simulink model "DEF_IEEE14_case1"  (R2023b)
settings: Solver=FixedStepAuto  StartTime=0  StopTime=80  FixedStep=Ts  RelTol=1e-3
StopFcn:
  | %data_idq_all = out.data_idq_all;
  | %save('Oscillation_July\data\data_idq_all.mat','data_idq_all');
  | %data_vdq_all = out.data_vdq_all;
  | %save('Oscillation_July\data\data_vdq_all.mat','data_vdq_all');
values from neighbouring files (symbols this model uses):
  freq_sel = imag(Mode_Hz)    [Mode_Right_Eig.m]
  Mode_Rad = D(ModeSel, ModeSel)    [Mode_Right_Eig.m]
undefined symbols (not defined in the file or in its folder): ApparatusDiscreDamping, ApparatusPara, ApparatusPowerFlow, ApparatusType, DiscIntNeverNeededParam, Fbase, fpll, k_lpf, lpf_A, lpf_B, lpf_C, lpf_D, OtherInputs, Sbase, Tdef_start, Ts, Vbase, Wbase, wc_lpf, x_e, Ybase, Zbase
libraries: spsFourierLib x50, SimplusGT x46, spsGroundLib x22, spsThreePhaseSeriesRLCBranchLib x20, spsThreePhaseParallelRLCBranchLib x14, spsThreePhaseTransformerTwoWindingsLib x3, eeGeneralControl x2, spspowerguiLib x1
(part 2 of 3)

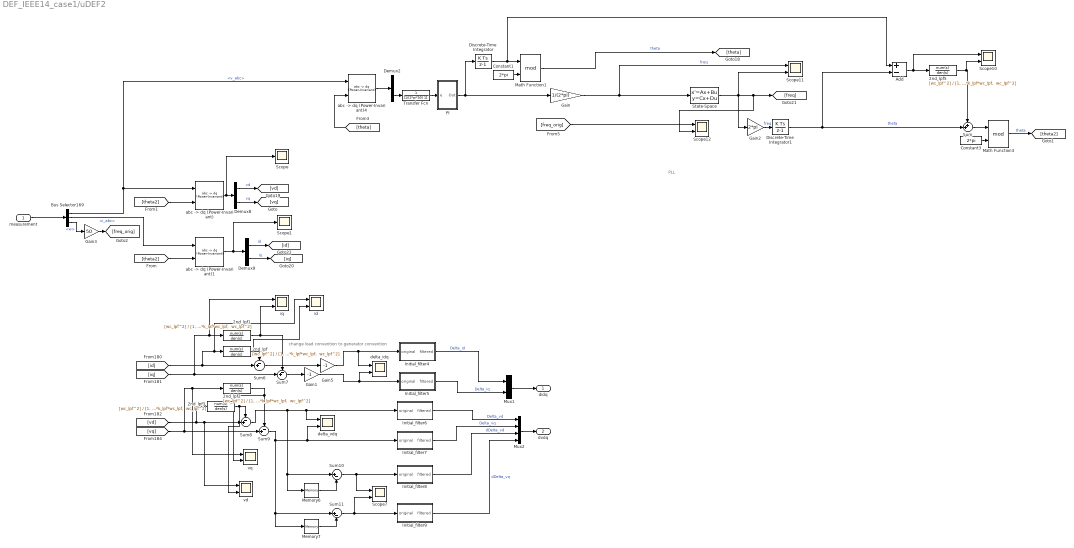
== system DEF_IEEE14_case1/uDEF2 ==
  note: change load convention to generator convention
  note: PLL
  measurement : Inport
  2nd_lpf{,1..3,5} (5 alike) : TransferFcn  Numerator=[wc_lpf^2]  Denominator="[1, 2*k_lpf*wc_lpf,  wc_lpf^2]"
  Add : Sum  Inputs=+-
  Bus Selector169 : BusSelector  OutputSignals=v_abc,i_abc,w
  Constant1 : Constant  Value=2*pi
  Constant3 : Constant  Value=2*pi
  Demux2 : Demux  Outputs=2
  Demux8 : Demux  Outputs=2
  Demux9 : Demux  Outputs=2
  Discrete-Time Integrator : DiscreteIntegrator  SampleTime=Ts  ICPrevOutput=DiscIntNeverNeededParam  ICPrevScaledInput=DiscIntNeverNeededParam
  Discrete-Time Integrator1 : DiscreteIntegrator  SampleTime=Ts  ICPrevOutput=DiscIntNeverNeededParam  ICPrevScaledInput=DiscIntNeverNeededParam
  Gain : Gain  Gain=1/(2*pi)
  Gain1 : Gain  Gain=-1
  Gain2 : Gain  Gain=2*pi
  Gain3 : Gain  Gain=50
  Gain5 : Gain  Gain=-1
  Initial_filter4 : Subsystem
  Initial_filter5 : Subsystem
  Initial_filter6 : Subsystem
  Initial_filter7 : Subsystem
  Initial_filter8 : Subsystem
  Initial_filter9 : Subsystem
  Math Function1 : Math  Operator=mod  SignedPower=on
  Math Function3 : Math  Operator=mod  SignedPower=on
  Memory6 : Memory
  Memory7 : Memory
  Mux1 : Mux  Inputs=2
  Mux2 : Mux
  PI : Subsystem  mask{Kp_PLL=2*pi*fpll, Ki_PLL=(2*pi*fpll)^2/4, IntSat_PLL=20000}
      mask prompts: Kp_PLL "Proportional (P)"; Ki_PLL "Integral (I)"; IntSat_PLL "Integrator Saturation Limit"
      mask DialogControl DescGroupVar Prompt: PLL Parameters
  Scope : Scope
  Scope1 : Scope
  Scope{7,10..12} (4 alike) : Scope  NumInputPorts=2
  State-Space : StateSpace  A=lpf_A  B=lpf_B  C=lpf_C  D=lpf_D  InitialCondition=[0,50/lpf_C(2)]
  Sum : Sum  Inputs=++|
  Sum10 : Sum  Inputs=|+-
  Sum11 : Sum  Inputs=|+-
  Sum{6..9} (4 alike) : Sum  Inputs=-+|
  Transfer Fcn : TransferFcn  Denominator=[1/(2*pi*50) 1]
  "abc -> dq (Power-Invariant)" : SimplusGT/abc -> dq (Power-Invariant)  SystemSampleTime=-1  VariantActivationTime=update diagram  AllowFlexibleInterface=on  Latency=0  AutoFrameSizeCalculation=off
      settings: SourceProductName=Simplus Grid Tool
  "abc -> dq (Power-Invariant)1" : SimplusGT/abc -> dq (Power-Invariant)  SystemSampleTime=-1  VariantActivationTime=update diagram  AllowFlexibleInterface=on  Latency=0  AutoFrameSizeCalculation=off
      settings: SourceProductName=Simplus Grid Tool
  "abc -> dq (Power-Invariant)4" : SimplusGT/abc -> dq (Power-Invariant)  SystemSampleTime=-1  VariantActivationTime=update diagram  AllowFlexibleInterface=on  Latency=0  AutoFrameSizeCalculation=off
      settings: SourceProductName=Simplus Grid Tool
  delta_idq : Scope  NumInputPorts=2
  delta_vdq : Scope  NumInputPorts=2
  id : Scope  NumInputPorts=2
  iq : Scope  NumInputPorts=2
  vd : Scope  NumInputPorts=2
  vq : Scope  NumInputPorts=2
  didq : Outport
  dvdq : Outport  Port=2
  wires:
  [vq] -> vq/1, 2nd_lpf2/1, Sum9/2
  Sum11/1 -> Scope7/2, Initial_filter9/1(original)
  Sum6/1 -> Gain5/1
  "abc -> dq (Power-Invariant)1"/1 -> Scope1/1, Demux9/1
  [theta2] -> "abc -> dq (Power-Invariant)1"/2
  Sum9/1 -> Memory7/1, Sum11/1, delta_vdq/2, Initial_filter7/1(original)
  [vd] -> 2nd_lpf3/1, vd/1, Sum8/2
  Demux9/1 -> [id]  "id"
  Sum8/1 -> Memory6/1, Sum10/1, delta_vdq/1, Initial_filter6/1(original)
  Initial_filter7/1(filtered) -> Mux2/2  "Delta_vq"
  Bus Selector169/1 -> "abc -> dq (Power-Invariant)4"/1, "abc -> dq (Power-Invariant)"/1  "<v_abc>"
  Demux9/2 -> [iq]  "iq"
  [id] -> id/1, 2nd_lpf/1, Sum6/2
  2nd_lpf/1 -> id/2, Sum6/1
  Sum10/1 -> Scope7/1, Initial_filter8/1(original)
  Memory7/1 -> Sum11/2
  Initial_filter9/1(filtered) -> Mux2/4  "dDelta_vq"
  2nd_lpf1/1 -> iq/2, Sum7/1
  Mux1/1 -> didq/1
  Memory6/1 -> Sum10/2
  Bus Selector169/2 -> "abc -> dq (Power-Invariant)1"/1  "<i_abc>"
  Sum7/1 -> Gain1/1
  Demux8/1 -> [vd]  "vd"
  Initial_filter6/1(filtered) -> Mux2/1  "Delta_vd"
  Initial_filter5/1(filtered) -> Mux1/2  "Delta_iq"
  Mux2/1 -> dvdq/1
  [iq] -> iq/1, 2nd_lpf1/1, Sum7/2
  Initial_filter4/1(filtered) -> Mux1/1  "Delta_id"
  2nd_lpf2/1 -> Sum9/1, vq/2
  Gain1/1 -> delta_idq/2, Initial_filter5/1(original)
  Demux8/2 -> [vq]  "vq"
  "abc -> dq (Power-Invariant)"/1 -> Scope/1, Demux8/1
  Initial_filter8/1(filtered) -> Mux2/3  "dDelta_vd"
  [theta2] -> "abc -> dq (Power-Invariant)"/2
  2nd_lpf3/1 -> vd/2, Sum8/1
  Gain5/1 -> delta_idq/1, Initial_filter4/1(original)
  [theta] -> "abc -> dq (Power-Invariant)4"/2
  Constant1/1 -> Math Function1/2
  Add/1 -> 2nd_lpf5/1, Scope10/1
  Discrete-Time Integrator/1 -> Math Function1/1, Add/1
  Gain2/1 -> Discrete-Time Integrator1/1  "freq"
  "abc -> dq (Power-Invariant)4"/1 -> Demux2/1
  Transfer Fcn/1 -> PI/1(e)
  Math Function1/1 -> [theta]  "theta"
  Gain/1 -> State-Space/1, Scope11/1  "freq"
  PI/1(Out) -> Gain/1, Discrete-Time Integrator/1
  Demux2/2 -> Transfer Fcn/1
  [freq_orig] -> Scope12/1
  Math Function3/1 -> [theta2]  "theta"
  2nd_lpf5/1 -> Sum/1, Scope10/2
  Sum/1 -> Math Function3/1
  State-Space/1 -> Scope12/2, [freq], Scope11/2, Gain2/1
  Constant3/1 -> Math Function3/2
  Discrete-Time Integrator1/1 -> Add/2, Sum/2  "theta"
  measurement/1 -> Bus Selector169/1
  Gain3/1 -> [freq_orig]
  Bus Selector169/3 -> Gain3/1  "<w>"

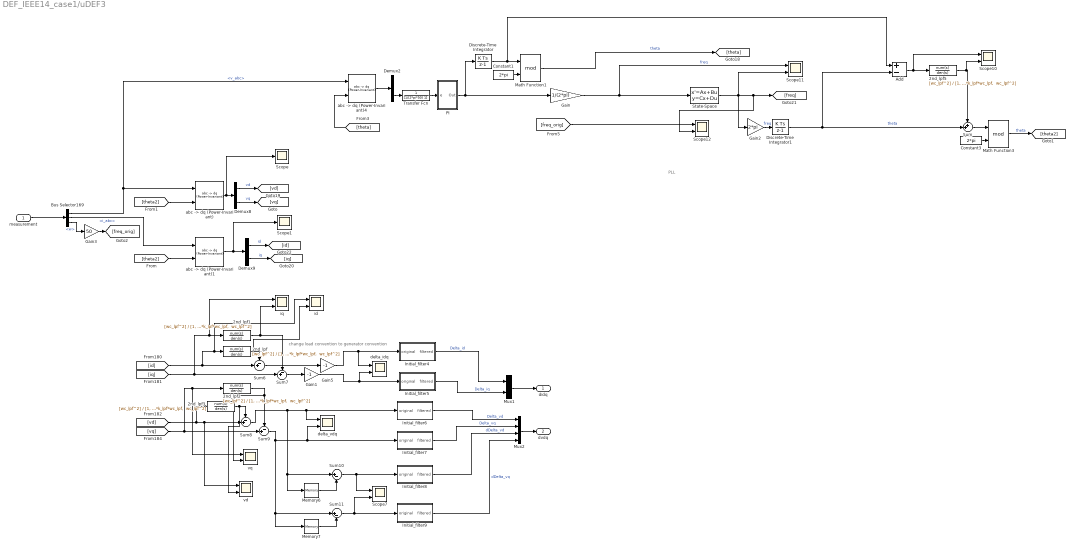
== system DEF_IEEE14_case1/uDEF3 ==
  note: PLL
  note: change load convention to generator convention
  measurement : Inport
  2nd_lpf{,1..3,5} (5 alike) : TransferFcn  Numerator=[wc_lpf^2]  Denominator="[1, 2*k_lpf*wc_lpf,  wc_lpf^2]"
  Add : Sum  Inputs=+-
  Bus Selector169 : BusSelector  OutputSignals=v_abc,i_abc,w
  Constant1 : Constant  Value=2*pi
  Constant3 : Constant  Value=2*pi
  Demux2 : Demux  Outputs=2
  Demux8 : Demux  Outputs=2
  Demux9 : Demux  Outputs=2
  Discrete-Time Integrator : DiscreteIntegrator  SampleTime=Ts  ICPrevOutput=DiscIntNeverNeededParam  ICPrevScaledInput=DiscIntNeverNeededParam
  Discrete-Time Integrator1 : DiscreteIntegrator  SampleTime=Ts  ICPrevOutput=DiscIntNeverNeededParam  ICPrevScaledInput=DiscIntNeverNeededParam
  Gain : Gain  Gain=1/(2*pi)
  Gain1 : Gain  Gain=-1
  Gain2 : Gain  Gain=2*pi
  Gain3 : Gain  Gain=50
  Gain5 : Gain  Gain=-1
  Initial_filter4 : Subsystem
  Initial_filter5 : Subsystem
  Initial_filter6 : Subsystem
  Initial_filter7 : Subsystem
  Initial_filter8 : Subsystem
  Initial_filter9 : Subsystem
  Math Function1 : Math  Operator=mod  SignedPower=on
  Math Function3 : Math  Operator=mod  SignedPower=on
  Memory6 : Memory
  Memory7 : Memory
  Mux1 : Mux  Inputs=2
  Mux2 : Mux
  PI : Subsystem  mask{Kp_PLL=2*pi*fpll, Ki_PLL=(2*pi*fpll)^2/4, IntSat_PLL=20000}
      mask prompts: Kp_PLL "Proportional (P)"; Ki_PLL "Integral (I)"; IntSat_PLL "Integrator Saturation Limit"
      mask DialogControl DescGroupVar Prompt: PLL Parameters
  Scope : Scope
  Scope1 : Scope
  Scope{7,10..12} (4 alike) : Scope  NumInputPorts=2
  State-Space : StateSpace  A=lpf_A  B=lpf_B  C=lpf_C  D=lpf_D  InitialCondition=[0,50/lpf_C(2)]
  Sum : Sum  Inputs=++|
  Sum10 : Sum  Inputs=|+-
  Sum11 : Sum  Inputs=|+-
  Sum{6..9} (4 alike) : Sum  Inputs=-+|
  Transfer Fcn : TransferFcn  Denominator=[1/(2*pi*50) 1]
  "abc -> dq (Power-Invariant)" : SimplusGT/abc -> dq (Power-Invariant)  SystemSampleTime=-1  VariantActivationTime=update diagram  AllowFlexibleInterface=on  Latency=0  AutoFrameSizeCalculation=off
      settings: SourceProductName=Simplus Grid Tool
  "abc -> dq (Power-Invariant)1" : SimplusGT/abc -> dq (Power-Invariant)  SystemSampleTime=-1  VariantActivationTime=update diagram  AllowFlexibleInterface=on  Latency=0  AutoFrameSizeCalculation=off
      settings: SourceProductName=Simplus Grid Tool
  "abc -> dq (Power-Invariant)4" : SimplusGT/abc -> dq (Power-Invariant)  SystemSampleTime=-1  VariantActivationTime=update diagram  AllowFlexibleInterface=on  Latency=0  AutoFrameSizeCalculation=off
      settings: SourceProductName=Simplus Grid Tool
  delta_idq : Scope  NumInputPorts=2
  delta_vdq : Scope  NumInputPorts=2
  id : Scope  NumInputPorts=2
  iq : Scope  NumInputPorts=2
  vd : Scope  NumInputPorts=2
  vq : Scope  NumInputPorts=2
  didq : Outport
  dvdq : Outport  Port=2
  wires:
  Bus Selector169/3 -> Gain3/1  "<w>"
  Gain3/1 -> [freq_orig]
  measurement/1 -> Bus Selector169/1
  Discrete-Time Integrator1/1 -> Sum/2, Add/2  "theta"
  Constant3/1 -> Math Function3/2
  State-Space/1 -> Gain2/1, Scope11/2, [freq], Scope12/2
  Sum/1 -> Math Function3/1
  2nd_lpf5/1 -> Scope10/2, Sum/1
  Math Function3/1 -> [theta2]  "theta"
  [freq_orig] -> Scope12/1
  Demux2/2 -> Transfer Fcn/1
  PI/1(Out) -> Discrete-Time Integrator/1, Gain/1
  Gain/1 -> Scope11/1, State-Space/1  "freq"
  Math Function1/1 -> [theta]  "theta"
  Transfer Fcn/1 -> PI/1(e)
  "abc -> dq (Power-Invariant)4"/1 -> Demux2/1
  Gain2/1 -> Discrete-Time Integrator1/1  "freq"
  Discrete-Time Integrator/1 -> Add/1, Math Function1/1
  Add/1 -> Scope10/1, 2nd_lpf5/1
  Constant1/1 -> Math Function1/2
  [theta] -> "abc -> dq (Power-Invariant)4"/2
  Gain5/1 -> Initial_filter4/1(original), delta_idq/1
  2nd_lpf3/1 -> Sum8/1, vd/2
  [theta2] -> "abc -> dq (Power-Invariant)"/2
  Initial_filter8/1(filtered) -> Mux2/3  "dDelta_vd"
  "abc -> dq (Power-Invariant)"/1 -> Demux8/1, Scope/1
  Demux8/2 -> [vq]  "vq"
  Gain1/1 -> Initial_filter5/1(original), delta_idq/2
  2nd_lpf2/1 -> vq/2, Sum9/1
  Initial_filter4/1(filtered) -> Mux1/1  "Delta_id"
  [iq] -> Sum7/2, 2nd_lpf1/1, iq/1
  Mux2/1 -> dvdq/1
  Initial_filter5/1(filtered) -> Mux1/2  "Delta_iq"
  Initial_filter6/1(filtered) -> Mux2/1  "Delta_vd"
  Demux8/1 -> [vd]  "vd"
  Sum7/1 -> Gain1/1
  Bus Selector169/2 -> "abc -> dq (Power-Invariant)1"/1  "<i_abc>"
  Memory6/1 -> Sum10/2
  Mux1/1 -> didq/1
  2nd_lpf1/1 -> Sum7/1, iq/2
  Initial_filter9/1(filtered) -> Mux2/4  "dDelta_vq"
  Memory7/1 -> Sum11/2
  Sum10/1 -> Initial_filter8/1(original), Scope7/1
  2nd_lpf/1 -> Sum6/1, id/2
  [id] -> Sum6/2, 2nd_lpf/1, id/1
  Demux9/2 -> [iq]  "iq"
  Bus Selector169/1 -> "abc -> dq (Power-Invariant)"/1, "abc -> dq (Power-Invariant)4"/1  "<v_abc>"
  Initial_filter7/1(filtered) -> Mux2/2  "Delta_vq"
  Sum8/1 -> Initial_filter6/1(original), delta_vdq/1, Sum10/1, Memory6/1
  Demux9/1 -> [id]  "id"
  [vd] -> Sum8/2, vd/1, 2nd_lpf3/1
  Sum9/1 -> Initial_filter7/1(original), delta_vdq/2, Sum11/1, Memory7/1
  [theta2] -> "abc -> dq (Power-Invariant)1"/2
  "abc -> dq (Power-Invariant)1"/1 -> Demux9/1, Scope1/1
  Sum6/1 -> Gain5/1
  Sum11/1 -> Initial_filter9/1(original), Scope7/2
  [vq] -> Sum9/2, 2nd_lpf2/1, vq/1

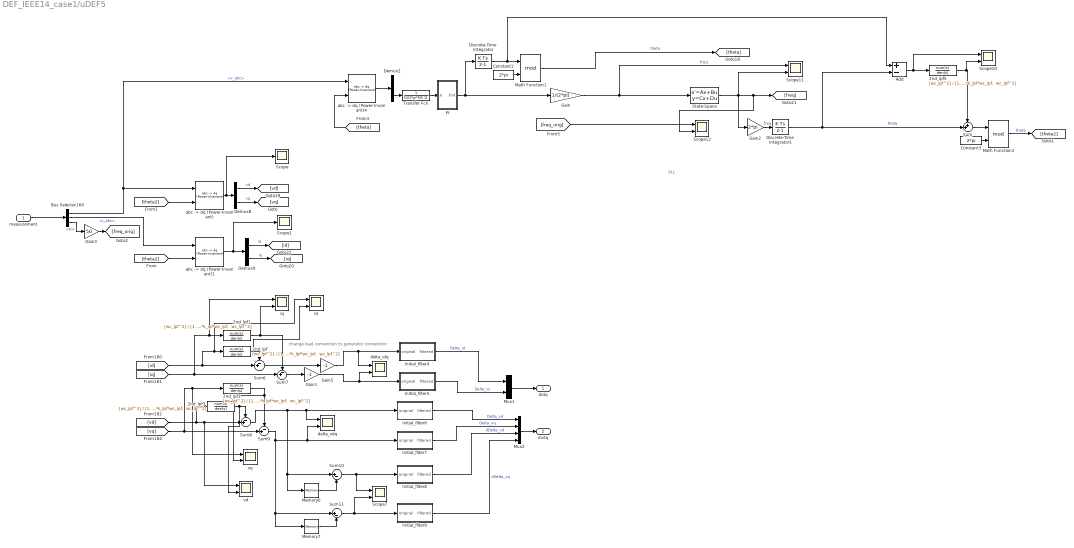
== system DEF_IEEE14_case1/uDEF5 ==
  note: change load convention to generator convention
  note: PLL
  measurement : Inport
  2nd_lpf{,1..3,5} (5 alike) : TransferFcn  Numerator=[wc_lpf^2]  Denominator="[1, 2*k_lpf*wc_lpf,  wc_lpf^2]"
  Add : Sum  Inputs=+-
  Bus Selector169 : BusSelector  OutputSignals=v_abc,i_abc,w
  Constant1 : Constant  Value=2*pi
  Constant3 : Constant  Value=2*pi
  Demux2 : Demux  Outputs=2
  Demux8 : Demux  Outputs=2
  Demux9 : Demux  Outputs=2
  Discrete-Time Integrator : DiscreteIntegrator  SampleTime=Ts  ICPrevOutput=DiscIntNeverNeededParam  ICPrevScaledInput=DiscIntNeverNeededParam
  Discrete-Time Integrator1 : DiscreteIntegrator  SampleTime=Ts  ICPrevOutput=DiscIntNeverNeededParam  ICPrevScaledInput=DiscIntNeverNeededParam
  Gain : Gain  Gain=1/(2*pi)
  Gain1 : Gain  Gain=-1
  Gain2 : Gain  Gain=2*pi
  Gain3 : Gain  Gain=50
  Gain5 : Gain  Gain=-1
  Initial_filter4 : Subsystem
  Initial_filter5 : Subsystem
  Initial_filter6 : Subsystem
  Initial_filter7 : Subsystem
  Initial_filter8 : Subsystem
  Initial_filter9 : Subsystem
  Math Function1 : Math  Operator=mod  SignedPower=on
  Math Function3 : Math  Operator=mod  SignedPower=on
  Memory6 : Memory
  Memory7 : Memory
  Mux1 : Mux  Inputs=2
  Mux2 : Mux
  PI : Subsystem  mask{Kp_PLL=2*pi*fpll, Ki_PLL=(2*pi*fpll)^2/4, IntSat_PLL=20000}
      mask prompts: Kp_PLL "Proportional (P)"; Ki_PLL "Integral (I)"; IntSat_PLL "Integrator Saturation Limit"
      mask DialogControl DescGroupVar Prompt: PLL Parameters
  Scope : Scope
  Scope1 : Scope
  Scope{7,10..12} (4 alike) : Scope  NumInputPorts=2
  State-Space : StateSpace  A=lpf_A  B=lpf_B  C=lpf_C  D=lpf_D  InitialCondition=[0,50/lpf_C(2)]
  Sum : Sum  Inputs=++|
  Sum10 : Sum  Inputs=|+-
  Sum11 : Sum  Inputs=|+-
  Sum{6..9} (4 alike) : Sum  Inputs=-+|
  Transfer Fcn : TransferFcn  Denominator=[1/(2*pi*50) 1]
  "abc -> dq (Power-Invariant)" : SimplusGT/abc -> dq (Power-Invariant)  SystemSampleTime=-1  VariantActivationTime=update diagram  AllowFlexibleInterface=on  Latency=0  AutoFrameSizeCalculation=off
      settings: SourceProductName=Simplus Grid Tool
  "abc -> dq (Power-Invariant)1" : SimplusGT/abc -> dq (Power-Invariant)  SystemSampleTime=-1  VariantActivationTime=update diagram  AllowFlexibleInterface=on  Latency=0  AutoFrameSizeCalculation=off
      settings: SourceProductName=Simplus Grid Tool
  "abc -> dq (Power-Invariant)4" : SimplusGT/abc -> dq (Power-Invariant)  SystemSampleTime=-1  VariantActivationTime=update diagram  AllowFlexibleInterface=on  Latency=0  AutoFrameSizeCalculation=off
      settings: SourceProductName=Simplus Grid Tool
  delta_idq : Scope  NumInputPorts=2
  delta_vdq : Scope  NumInputPorts=2
  id : Scope  NumInputPorts=2
  iq : Scope  NumInputPorts=2
  vd : Scope  NumInputPorts=2
  vq : Scope  NumInputPorts=2
  didq : Outport
  dvdq : Outport  Port=2
  wires:
  [vq] -> vq/1, 2nd_lpf2/1, Sum9/2
  Sum11/1 -> Scope7/2, Initial_filter9/1(original)
  Sum6/1 -> Gain5/1
  "abc -> dq (Power-Invariant)1"/1 -> Scope1/1, Demux9/1
  [theta2] -> "abc -> dq (Power-Invariant)1"/2
  Sum9/1 -> Memory7/1, Sum11/1, delta_vdq/2, Initial_filter7/1(original)
  [vd] -> 2nd_lpf3/1, vd/1, Sum8/2
  Demux9/1 -> [id]  "id"
  Sum8/1 -> Memory6/1, Sum10/1, delta_vdq/1, Initial_filter6/1(original)
  Initial_filter7/1(filtered) -> Mux2/2  "Delta_vq"
  Bus Selector169/1 -> "abc -> dq (Power-Invariant)4"/1, "abc -> dq (Power-Invariant)"/1  "<v_abc>"
  Demux9/2 -> [iq]  "iq"
  [id] -> id/1, 2nd_lpf/1, Sum6/2
  2nd_lpf/1 -> id/2, Sum6/1
  Sum10/1 -> Scope7/1, Initial_filter8/1(original)
  Memory7/1 -> Sum11/2
  Initial_filter9/1(filtered) -> Mux2/4  "dDelta_vq"
  2nd_lpf1/1 -> iq/2, Sum7/1
  Mux1/1 -> didq/1
  Memory6/1 -> Sum10/2
  Bus Selector169/2 -> "abc -> dq (Power-Invariant)1"/1  "<i_abc>"
  Sum7/1 -> Gain1/1
  Demux8/1 -> [vd]  "vd"
  Initial_filter6/1(filtered) -> Mux2/1  "Delta_vd"
  Initial_filter5/1(filtered) -> Mux1/2  "Delta_iq"
  Mux2/1 -> dvdq/1
  [iq] -> iq/1, 2nd_lpf1/1, Sum7/2
  Initial_filter4/1(filtered) -> Mux1/1  "Delta_id"
  2nd_lpf2/1 -> Sum9/1, vq/2
  Gain1/1 -> delta_idq/2, Initial_filter5/1(original)
  Demux8/2 -> [vq]  "vq"
  "abc -> dq (Power-Invariant)"/1 -> Scope/1, Demux8/1
  Initial_filter8/1(filtered) -> Mux2/3  "dDelta_vd"
  [theta2] -> "abc -> dq (Power-Invariant)"/2
  2nd_lpf3/1 -> vd/2, Sum8/1
  Gain5/1 -> delta_idq/1, Initial_filter4/1(original)
  [theta] -> "abc -> dq (Power-Invariant)4"/2
  Constant1/1 -> Math Function1/2
  Add/1 -> 2nd_lpf5/1, Scope10/1
  Discrete-Time Integrator/1 -> Math Function1/1, Add/1
  Gain2/1 -> Discrete-Time Integrator1/1  "freq"
  "abc -> dq (Power-Invariant)4"/1 -> Demux2/1
  Transfer Fcn/1 -> PI/1(e)
  Math Function1/1 -> [theta]  "theta"
  Gain/1 -> State-Space/1, Scope11/1  "freq"
  PI/1(Out) -> Gain/1, Discrete-Time Integrator/1
  Demux2/2 -> Transfer Fcn/1
  [freq_orig] -> Scope12/1
  Math Function3/1 -> [theta2]  "theta"
  2nd_lpf5/1 -> Sum/1, Scope10/2
  Sum/1 -> Math Function3/1
  State-Space/1 -> Scope12/2, [freq], Scope11/2, Gain2/1
  Constant3/1 -> Math Function3/2
  Discrete-Time Integrator1/1 -> Add/2, Sum/2  "theta"
  measurement/1 -> Bus Selector169/1
  Gain3/1 -> [freq_orig]
  Bus Selector169/3 -> Gain3/1  "<w>"

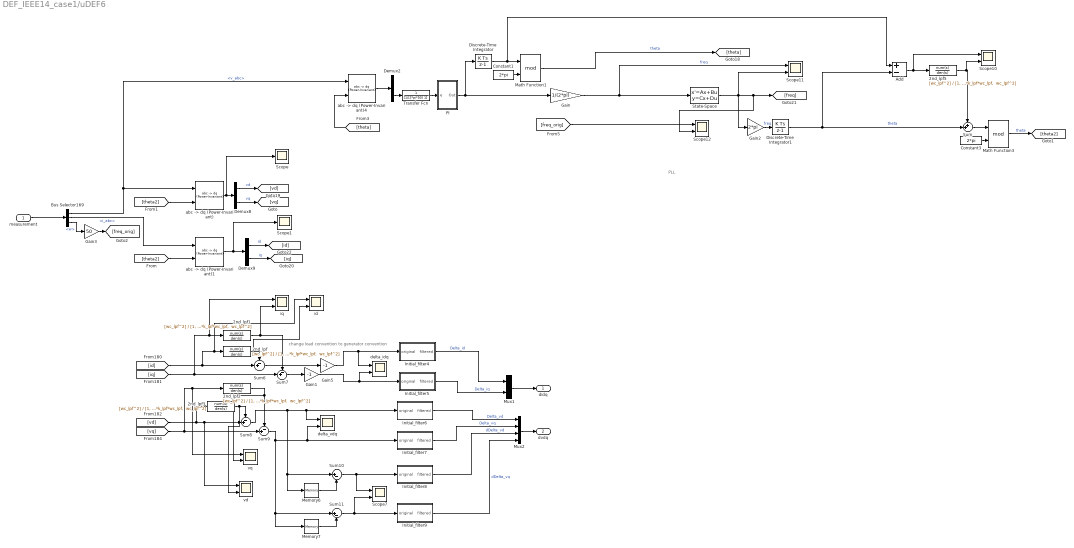
== system DEF_IEEE14_case1/uDEF6 ==
  note: PLL
  note: change load convention to generator convention
  measurement : Inport
  2nd_lpf{,1..3,5} (5 alike) : TransferFcn  Numerator=[wc_lpf^2]  Denominator="[1, 2*k_lpf*wc_lpf,  wc_lpf^2]"
  Add : Sum  Inputs=+-
  Bus Selector169 : BusSelector  OutputSignals=v_abc,i_abc,w
  Constant1 : Constant  Value=2*pi
  Constant3 : Constant  Value=2*pi
  Demux2 : Demux  Outputs=2
  Demux8 : Demux  Outputs=2
  Demux9 : Demux  Outputs=2
  Discrete-Time Integrator : DiscreteIntegrator  SampleTime=Ts  ICPrevOutput=DiscIntNeverNeededParam  ICPrevScaledInput=DiscIntNeverNeededParam
  Discrete-Time Integrator1 : DiscreteIntegrator  SampleTime=Ts  ICPrevOutput=DiscIntNeverNeededParam  ICPrevScaledInput=DiscIntNeverNeededParam
  Gain : Gain  Gain=1/(2*pi)
  Gain1 : Gain  Gain=-1
  Gain2 : Gain  Gain=2*pi
  Gain3 : Gain  Gain=50
  Gain5 : Gain  Gain=-1
  Initial_filter4 : Subsystem
  Initial_filter5 : Subsystem
  Initial_filter6 : Subsystem
  Initial_filter7 : Subsystem
  Initial_filter8 : Subsystem
  Initial_filter9 : Subsystem
  Math Function1 : Math  Operator=mod  SignedPower=on
  Math Function3 : Math  Operator=mod  SignedPower=on
  Memory6 : Memory
  Memory7 : Memory
  Mux1 : Mux  Inputs=2
  Mux2 : Mux
  PI : Subsystem  mask{Kp_PLL=2*pi*fpll, Ki_PLL=(2*pi*fpll)^2/4, IntSat_PLL=20000}
      mask prompts: Kp_PLL "Proportional (P)"; Ki_PLL "Integral (I)"; IntSat_PLL "Integrator Saturation Limit"
      mask DialogControl DescGroupVar Prompt: PLL Parameters
  Scope : Scope
  Scope1 : Scope
  Scope{7,10..12} (4 alike) : Scope  NumInputPorts=2
  State-Space : StateSpace  A=lpf_A  B=lpf_B  C=lpf_C  D=lpf_D  InitialCondition=[0,50/lpf_C(2)]
  Sum : Sum  Inputs=++|
  Sum10 : Sum  Inputs=|+-
  Sum11 : Sum  Inputs=|+-
  Sum{6..9} (4 alike) : Sum  Inputs=-+|
  Transfer Fcn : TransferFcn  Denominator=[1/(2*pi*50) 1]
  "abc -> dq (Power-Invariant)" : SimplusGT/abc -> dq (Power-Invariant)  SystemSampleTime=-1  VariantActivationTime=update diagram  AllowFlexibleInterface=on  Latency=0  AutoFrameSizeCalculation=off
      settings: SourceProductName=Simplus Grid Tool
  "abc -> dq (Power-Invariant)1" : SimplusGT/abc -> dq (Power-Invariant)  SystemSampleTime=-1  VariantActivationTime=update diagram  AllowFlexibleInterface=on  Latency=0  AutoFrameSizeCalculation=off
      settings: SourceProductName=Simplus Grid Tool
  "abc -> dq (Power-Invariant)4" : SimplusGT/abc -> dq (Power-Invariant)  SystemSampleTime=-1  VariantActivationTime=update diagram  AllowFlexibleInterface=on  Latency=0  AutoFrameSizeCalculation=off
      settings: SourceProductName=Simplus Grid Tool
  delta_idq : Scope  NumInputPorts=2
  delta_vdq : Scope  NumInputPorts=2
  id : Scope  NumInputPorts=2
  iq : Scope  NumInputPorts=2
  vd : Scope  NumInputPorts=2
  vq : Scope  NumInputPorts=2
  didq : Outport
  dvdq : Outport  Port=2
  wires:
  Bus Selector169/3 -> Gain3/1  "<w>"
  Gain3/1 -> [freq_orig]
  measurement/1 -> Bus Selector169/1
  Discrete-Time Integrator1/1 -> Sum/2, Add/2  "theta"
  Constant3/1 -> Math Function3/2
  State-Space/1 -> Gain2/1, Scope11/2, [freq], Scope12/2
  Sum/1 -> Math Function3/1
  2nd_lpf5/1 -> Scope10/2, Sum/1
  Math Function3/1 -> [theta2]  "theta"
  [freq_orig] -> Scope12/1
  Demux2/2 -> Transfer Fcn/1
  PI/1(Out) -> Discrete-Time Integrator/1, Gain/1
  Gain/1 -> Scope11/1, State-Space/1  "freq"
  Math Function1/1 -> [theta]  "theta"
  Transfer Fcn/1 -> PI/1(e)
  "abc -> dq (Power-Invariant)4"/1 -> Demux2/1
  Gain2/1 -> Discrete-Time Integrator1/1  "freq"
  Discrete-Time Integrator/1 -> Add/1, Math Function1/1
  Add/1 -> Scope10/1, 2nd_lpf5/1
  Constant1/1 -> Math Function1/2
  [theta] -> "abc -> dq (Power-Invariant)4"/2
  Gain5/1 -> Initial_filter4/1(original), delta_idq/1
  2nd_lpf3/1 -> Sum8/1, vd/2
  [theta2] -> "abc -> dq (Power-Invariant)"/2
  Initial_filter8/1(filtered) -> Mux2/3  "dDelta_vd"
  "abc -> dq (Power-Invariant)"/1 -> Demux8/1, Scope/1
  Demux8/2 -> [vq]  "vq"
  Gain1/1 -> Initial_filter5/1(original), delta_idq/2
  2nd_lpf2/1 -> vq/2, Sum9/1
  Initial_filter4/1(filtered) -> Mux1/1  "Delta_id"
  [iq] -> Sum7/2, 2nd_lpf1/1, iq/1
  Mux2/1 -> dvdq/1
  Initial_filter5/1(filtered) -> Mux1/2  "Delta_iq"
  Initial_filter6/1(filtered) -> Mux2/1  "Delta_vd"
  Demux8/1 -> [vd]  "vd"
  Sum7/1 -> Gain1/1
  Bus Selector169/2 -> "abc -> dq (Power-Invariant)1"/1  "<i_abc>"
  Memory6/1 -> Sum10/2
  Mux1/1 -> didq/1
  2nd_lpf1/1 -> Sum7/1, iq/2
  Initial_filter9/1(filtered) -> Mux2/4  "dDelta_vq"
  Memory7/1 -> Sum11/2
  Sum10/1 -> Initial_filter8/1(original), Scope7/1
  2nd_lpf/1 -> Sum6/1, id/2
  [id] -> Sum6/2, 2nd_lpf/1, id/1
  Demux9/2 -> [iq]  "iq"
  Bus Selector169/1 -> "abc -> dq (Power-Invariant)"/1, "abc -> dq (Power-Invariant)4"/1  "<v_abc>"
  Initial_filter7/1(filtered) -> Mux2/2  "Delta_vq"
  Sum8/1 -> Initial_filter6/1(original), delta_vdq/1, Sum10/1, Memory6/1
  Demux9/1 -> [id]  "id"
  [vd] -> Sum8/2, vd/1, 2nd_lpf3/1
  Sum9/1 -> Initial_filter7/1(original), delta_vdq/2, Sum11/1, Memory7/1
  [theta2] -> "abc -> dq (Power-Invariant)1"/2
  "abc -> dq (Power-Invariant)1"/1 -> Demux9/1, Scope1/1
  Sum6/1 -> Gain5/1
  Sum11/1 -> Initial_filter9/1(original), Scope7/2
  [vq] -> Sum9/2, 2nd_lpf2/1, vq/1

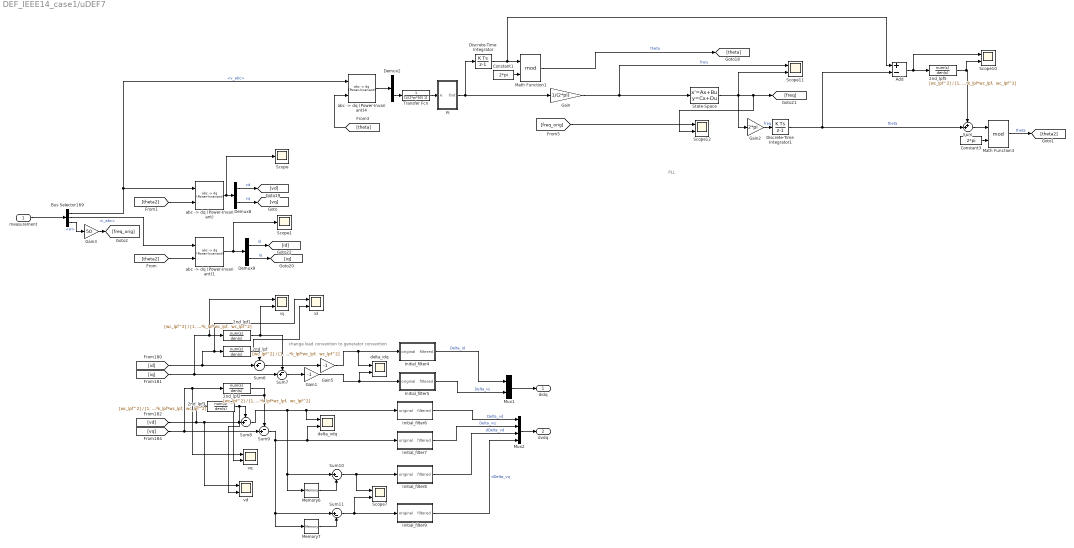
== system DEF_IEEE14_case1/uDEF7 ==
  note: change load convention to generator convention
  note: PLL
  measurement : Inport
  2nd_lpf{,1..3,5} (5 alike) : TransferFcn  Numerator=[wc_lpf^2]  Denominator="[1, 2*k_lpf*wc_lpf,  wc_lpf^2]"
  Add : Sum  Inputs=+-
  Bus Selector169 : BusSelector  OutputSignals=v_abc,i_abc,w
  Constant1 : Constant  Value=2*pi
  Constant3 : Constant  Value=2*pi
  Demux2 : Demux  Outputs=2
  Demux8 : Demux  Outputs=2
  Demux9 : Demux  Outputs=2
  Discrete-Time Integrator : DiscreteIntegrator  SampleTime=Ts  ICPrevOutput=DiscIntNeverNeededParam  ICPrevScaledInput=DiscIntNeverNeededParam
  Discrete-Time Integrator1 : DiscreteIntegrator  SampleTime=Ts  ICPrevOutput=DiscIntNeverNeededParam  ICPrevScaledInput=DiscIntNeverNeededParam
  Gain : Gain  Gain=1/(2*pi)
  Gain1 : Gain  Gain=-1
  Gain2 : Gain  Gain=2*pi
  Gain3 : Gain  Gain=50
  Gain5 : Gain  Gain=-1
  Initial_filter4 : Subsystem
  Initial_filter5 : Subsystem
  Initial_filter6 : Subsystem
  Initial_filter7 : Subsystem
  Initial_filter8 : Subsystem
  Initial_filter9 : Subsystem
  Math Function1 : Math  Operator=mod  SignedPower=on
  Math Function3 : Math  Operator=mod  SignedPower=on
  Memory6 : Memory
  Memory7 : Memory
  Mux1 : Mux  Inputs=2
  Mux2 : Mux
  PI : Subsystem  mask{Kp_PLL=2*pi*fpll, Ki_PLL=(2*pi*fpll)^2/4, IntSat_PLL=20000}
      mask prompts: Kp_PLL "Proportional (P)"; Ki_PLL "Integral (I)"; IntSat_PLL "Integrator Saturation Limit"
      mask DialogControl DescGroupVar Prompt: PLL Parameters
  Scope : Scope
  Scope1 : Scope
  Scope{7,10..12} (4 alike) : Scope  NumInputPorts=2
  State-Space : StateSpace  A=lpf_A  B=lpf_B  C=lpf_C  D=lpf_D  InitialCondition=[0,50/lpf_C(2)]
  Sum : Sum  Inputs=++|
  Sum10 : Sum  Inputs=|+-
  Sum11 : Sum  Inputs=|+-
  Sum{6..9} (4 alike) : Sum  Inputs=-+|
  Transfer Fcn : TransferFcn  Denominator=[1/(2*pi*50) 1]
  "abc -> dq (Power-Invariant)" : SimplusGT/abc -> dq (Power-Invariant)  SystemSampleTime=-1  VariantActivationTime=update diagram  AllowFlexibleInterface=on  Latency=0  AutoFrameSizeCalculation=off
      settings: SourceProductName=Simplus Grid Tool
  "abc -> dq (Power-Invariant)1" : SimplusGT/abc -> dq (Power-Invariant)  SystemSampleTime=-1  VariantActivationTime=update diagram  AllowFlexibleInterface=on  Latency=0  AutoFrameSizeCalculation=off
      settings: SourceProductName=Simplus Grid Tool
  "abc -> dq (Power-Invariant)4" : SimplusGT/abc -> dq (Power-Invariant)  SystemSampleTime=-1  VariantActivationTime=update diagram  AllowFlexibleInterface=on  Latency=0  AutoFrameSizeCalculation=off
      settings: SourceProductName=Simplus Grid Tool
  delta_idq : Scope  NumInputPorts=2
  delta_vdq : Scope  NumInputPorts=2
  id : Scope  NumInputPorts=2
  iq : Scope  NumInputPorts=2
  vd : Scope  NumInputPorts=2
  vq : Scope  NumInputPorts=2
  didq : Outport
  dvdq : Outport  Port=2
  wires:
  [vq] -> vq/1, 2nd_lpf2/1, Sum9/2
  Sum11/1 -> Scope7/2, Initial_filter9/1(original)
  Sum6/1 -> Gain5/1
  "abc -> dq (Power-Invariant)1"/1 -> Scope1/1, Demux9/1
  [theta2] -> "abc -> dq (Power-Invariant)1"/2
  Sum9/1 -> Memory7/1, Sum11/1, delta_vdq/2, Initial_filter7/1(original)
  [vd] -> 2nd_lpf3/1, vd/1, Sum8/2
  Demux9/1 -> [id]  "id"
  Sum8/1 -> Memory6/1, Sum10/1, delta_vdq/1, Initial_filter6/1(original)
  Initial_filter7/1(filtered) -> Mux2/2  "Delta_vq"
  Bus Selector169/1 -> "abc -> dq (Power-Invariant)4"/1, "abc -> dq (Power-Invariant)"/1  "<v_abc>"
  Demux9/2 -> [iq]  "iq"
  [id] -> id/1, 2nd_lpf/1, Sum6/2
  2nd_lpf/1 -> id/2, Sum6/1
  Sum10/1 -> Scope7/1, Initial_filter8/1(original)
  Memory7/1 -> Sum11/2
  Initial_filter9/1(filtered) -> Mux2/4  "dDelta_vq"
  2nd_lpf1/1 -> iq/2, Sum7/1
  Mux1/1 -> didq/1
  Memory6/1 -> Sum10/2
  Bus Selector169/2 -> "abc -> dq (Power-Invariant)1"/1  "<i_abc>"
  Sum7/1 -> Gain1/1
  Demux8/1 -> [vd]  "vd"
  Initial_filter6/1(filtered) -> Mux2/1  "Delta_vd"
  Initial_filter5/1(filtered) -> Mux1/2  "Delta_iq"
  Mux2/1 -> dvdq/1
  [iq] -> iq/1, 2nd_lpf1/1, Sum7/2
  Initial_filter4/1(filtered) -> Mux1/1  "Delta_id"
  2nd_lpf2/1 -> Sum9/1, vq/2
  Gain1/1 -> delta_idq/2, Initial_filter5/1(original)
  Demux8/2 -> [vq]  "vq"
  "abc -> dq (Power-Invariant)"/1 -> Scope/1, Demux8/1
  Initial_filter8/1(filtered) -> Mux2/3  "dDelta_vd"
  [theta2] -> "abc -> dq (Power-Invariant)"/2
  2nd_lpf3/1 -> vd/2, Sum8/1
  Gain5/1 -> delta_idq/1, Initial_filter4/1(original)
  [theta] -> "abc -> dq (Power-Invariant)4"/2
  Constant1/1 -> Math Function1/2
  Add/1 -> 2nd_lpf5/1, Scope10/1
  Discrete-Time Integrator/1 -> Math Function1/1, Add/1
  Gain2/1 -> Discrete-Time Integrator1/1  "freq"
  "abc -> dq (Power-Invariant)4"/1 -> Demux2/1
  Transfer Fcn/1 -> PI/1(e)
  Math Function1/1 -> [theta]  "theta"
  Gain/1 -> State-Space/1, Scope11/1  "freq"
  PI/1(Out) -> Gain/1, Discrete-Time Integrator/1
  Demux2/2 -> Transfer Fcn/1
  [freq_orig] -> Scope12/1
  Math Function3/1 -> [theta2]  "theta"
  2nd_lpf5/1 -> Sum/1, Scope10/2
  Sum/1 -> Math Function3/1
  State-Space/1 -> Scope12/2, [freq], Scope11/2, Gain2/1
  Constant3/1 -> Math Function3/2
  Discrete-Time Integrator1/1 -> Add/2, Sum/2  "theta"
  measurement/1 -> Bus Selector169/1
  Gain3/1 -> [freq_orig]
  Bus Selector169/3 -> Gain3/1  "<w>"

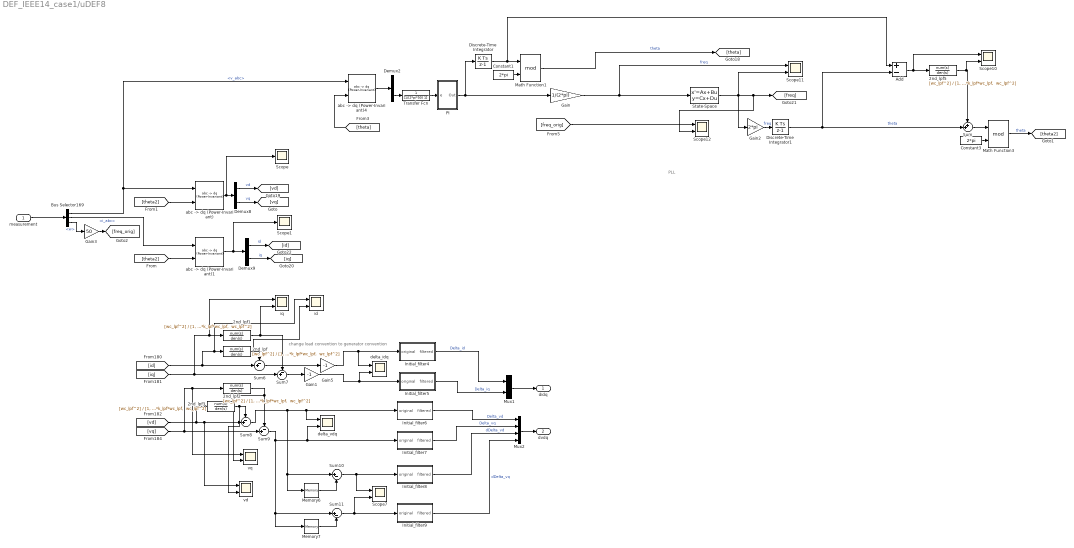
== system DEF_IEEE14_case1/uDEF8 ==
  note: PLL
  note: change load convention to generator convention
  measurement : Inport
  2nd_lpf{,1..3,5} (5 alike) : TransferFcn  Numerator=[wc_lpf^2]  Denominator="[1, 2*k_lpf*wc_lpf,  wc_lpf^2]"
  Add : Sum  Inputs=+-
  Bus Selector169 : BusSelector  OutputSignals=v_abc,i_abc,w
  Constant1 : Constant  Value=2*pi
  Constant3 : Constant  Value=2*pi
  Demux2 : Demux  Outputs=2
  Demux8 : Demux  Outputs=2
  Demux9 : Demux  Outputs=2
  Discrete-Time Integrator : DiscreteIntegrator  SampleTime=Ts  ICPrevOutput=DiscIntNeverNeededParam  ICPrevScaledInput=DiscIntNeverNeededParam
  Discrete-Time Integrator1 : DiscreteIntegrator  SampleTime=Ts  ICPrevOutput=DiscIntNeverNeededParam  ICPrevScaledInput=DiscIntNeverNeededParam
  Gain : Gain  Gain=1/(2*pi)
  Gain1 : Gain  Gain=-1
  Gain2 : Gain  Gain=2*pi
  Gain3 : Gain  Gain=50
  Gain5 : Gain  Gain=-1
  Initial_filter4 : Subsystem
  Initial_filter5 : Subsystem
  Initial_filter6 : Subsystem
  Initial_filter7 : Subsystem
  Initial_filter8 : Subsystem
  Initial_filter9 : Subsystem
  Math Function1 : Math  Operator=mod  SignedPower=on
  Math Function3 : Math  Operator=mod  SignedPower=on
  Memory6 : Memory
  Memory7 : Memory
  Mux1 : Mux  Inputs=2
  Mux2 : Mux
  PI : Subsystem  mask{Kp_PLL=2*pi*fpll, Ki_PLL=(2*pi*fpll)^2/4, IntSat_PLL=20000}
      mask prompts: Kp_PLL "Proportional (P)"; Ki_PLL "Integral (I)"; IntSat_PLL "Integrator Saturation Limit"
      mask DialogControl DescGroupVar Prompt: PLL Parameters
  Scope : Scope
  Scope1 : Scope
  Scope{7,10..12} (4 alike) : Scope  NumInputPorts=2
  State-Space : StateSpace  A=lpf_A  B=lpf_B  C=lpf_C  D=lpf_D  InitialCondition=[0,50/lpf_C(2)]
  Sum : Sum  Inputs=++|
  Sum10 : Sum  Inputs=|+-
  Sum11 : Sum  Inputs=|+-
  Sum{6..9} (4 alike) : Sum  Inputs=-+|
  Transfer Fcn : TransferFcn  Denominator=[1/(2*pi*50) 1]
  "abc -> dq (Power-Invariant)" : SimplusGT/abc -> dq (Power-Invariant)  SystemSampleTime=-1  VariantActivationTime=update diagram  AllowFlexibleInterface=on  Latency=0  AutoFrameSizeCalculation=off
      settings: SourceProductName=Simplus Grid Tool
  "abc -> dq (Power-Invariant)1" : SimplusGT/abc -> dq (Power-Invariant)  SystemSampleTime=-1  VariantActivationTime=update diagram  AllowFlexibleInterface=on  Latency=0  AutoFrameSizeCalculation=off
      settings: SourceProductName=Simplus Grid Tool
  "abc -> dq (Power-Invariant)4" : SimplusGT/abc -> dq (Power-Invariant)  SystemSampleTime=-1  VariantActivationTime=update diagram  AllowFlexibleInterface=on  Latency=0  AutoFrameSizeCalculation=off
      settings: SourceProductName=Simplus Grid Tool
  delta_idq : Scope  NumInputPorts=2
  delta_vdq : Scope  NumInputPorts=2
  id : Scope  NumInputPorts=2
  iq : Scope  NumInputPorts=2
  vd : Scope  NumInputPorts=2
  vq : Scope  NumInputPorts=2
  didq : Outport
  dvdq : Outport  Port=2
  wires:
  Bus Selector169/3 -> Gain3/1  "<w>"
  Gain3/1 -> [freq_orig]
  measurement/1 -> Bus Selector169/1
  Discrete-Time Integrator1/1 -> Sum/2, Add/2  "theta"
  Constant3/1 -> Math Function3/2
  State-Space/1 -> Gain2/1, Scope11/2, [freq], Scope12/2
  Sum/1 -> Math Function3/1
  2nd_lpf5/1 -> Scope10/2, Sum/1
  Math Function3/1 -> [theta2]  "theta"
  [freq_orig] -> Scope12/1
  Demux2/2 -> Transfer Fcn/1
  PI/1(Out) -> Discrete-Time Integrator/1, Gain/1
  Gain/1 -> Scope11/1, State-Space/1  "freq"
  Math Function1/1 -> [theta]  "theta"
  Transfer Fcn/1 -> PI/1(e)
  "abc -> dq (Power-Invariant)4"/1 -> Demux2/1
  Gain2/1 -> Discrete-Time Integrator1/1  "freq"
  Discrete-Time Integrator/1 -> Add/1, Math Function1/1
  Add/1 -> Scope10/1, 2nd_lpf5/1
  Constant1/1 -> Math Function1/2
  [theta] -> "abc -> dq (Power-Invariant)4"/2
  Gain5/1 -> Initial_filter4/1(original), delta_idq/1
  2nd_lpf3/1 -> Sum8/1, vd/2
  [theta2] -> "abc -> dq (Power-Invariant)"/2
  Initial_filter8/1(filtered) -> Mux2/3  "dDelta_vd"
  "abc -> dq (Power-Invariant)"/1 -> Demux8/1, Scope/1
  Demux8/2 -> [vq]  "vq"
  Gain1/1 -> Initial_filter5/1(original), delta_idq/2
  2nd_lpf2/1 -> vq/2, Sum9/1
  Initial_filter4/1(filtered) -> Mux1/1  "Delta_id"
  [iq] -> Sum7/2, 2nd_lpf1/1, iq/1
  Mux2/1 -> dvdq/1
  Initial_filter5/1(filtered) -> Mux1/2  "Delta_iq"
  Initial_filter6/1(filtered) -> Mux2/1  "Delta_vd"
  Demux8/1 -> [vd]  "vd"
  Sum7/1 -> Gain1/1
  Bus Selector169/2 -> "abc -> dq (Power-Invariant)1"/1  "<i_abc>"
  Memory6/1 -> Sum10/2
  Mux1/1 -> didq/1
  2nd_lpf1/1 -> Sum7/1, iq/2
  Initial_filter9/1(filtered) -> Mux2/4  "dDelta_vq"
  Memory7/1 -> Sum11/2
  Sum10/1 -> Initial_filter8/1(original), Scope7/1
  2nd_lpf/1 -> Sum6/1, id/2
  [id] -> Sum6/2, 2nd_lpf/1, id/1
  Demux9/2 -> [iq]  "iq"
  Bus Selector169/1 -> "abc -> dq (Power-Invariant)"/1, "abc -> dq (Power-Invariant)4"/1  "<v_abc>"
  Initial_filter7/1(filtered) -> Mux2/2  "Delta_vq"
  Sum8/1 -> Initial_filter6/1(original), delta_vdq/1, Sum10/1, Memory6/1
  Demux9/1 -> [id]  "id"
  [vd] -> Sum8/2, vd/1, 2nd_lpf3/1
  Sum9/1 -> Initial_filter7/1(original), delta_vdq/2, Sum11/1, Memory7/1
  [theta2] -> "abc -> dq (Power-Invariant)1"/2
  "abc -> dq (Power-Invariant)1"/1 -> Demux9/1, Scope1/1
  Sum6/1 -> Gain5/1
  Sum11/1 -> Initial_filter9/1(original), Scope7/2
  [vq] -> Sum9/2, 2nd_lpf2/1, vq/1

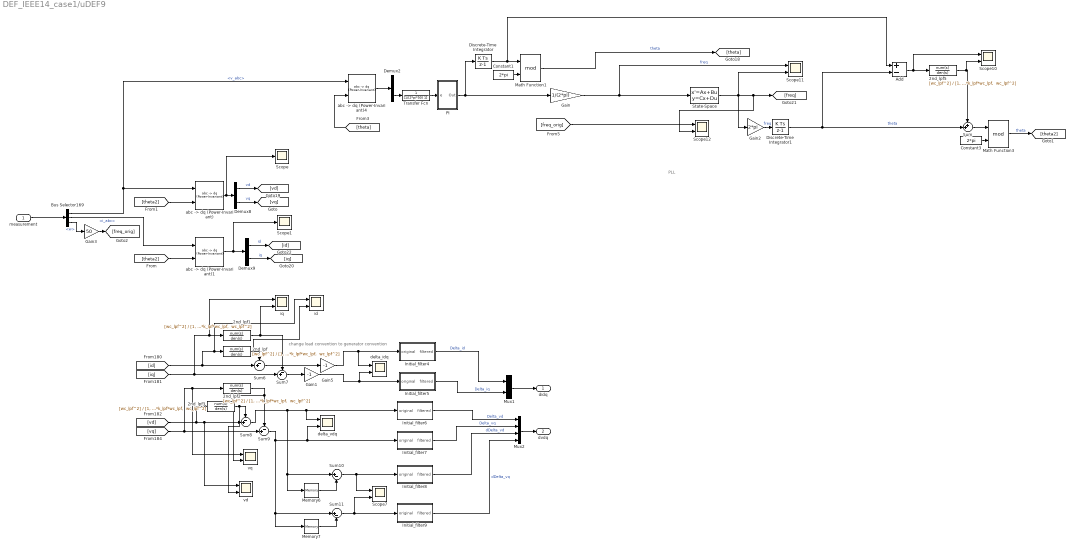
== system DEF_IEEE14_case1/uDEF9 ==
  note: change load convention to generator convention
  note: PLL
  measurement : Inport
  2nd_lpf{,1..3,5} (5 alike) : TransferFcn  Numerator=[wc_lpf^2]  Denominator="[1, 2*k_lpf*wc_lpf,  wc_lpf^2]"
  Add : Sum  Inputs=+-
  Bus Selector169 : BusSelector  OutputSignals=v_abc,i_abc,w
  Constant1 : Constant  Value=2*pi
  Constant3 : Constant  Value=2*pi
  Demux2 : Demux  Outputs=2
  Demux8 : Demux  Outputs=2
  Demux9 : Demux  Outputs=2
  Discrete-Time Integrator : DiscreteIntegrator  SampleTime=Ts  ICPrevOutput=DiscIntNeverNeededParam  ICPrevScaledInput=DiscIntNeverNeededParam
  Discrete-Time Integrator1 : DiscreteIntegrator  SampleTime=Ts  ICPrevOutput=DiscIntNeverNeededParam  ICPrevScaledInput=DiscIntNeverNeededParam
  Gain : Gain  Gain=1/(2*pi)
  Gain1 : Gain  Gain=-1
  Gain2 : Gain  Gain=2*pi
  Gain3 : Gain  Gain=50
  Gain5 : Gain  Gain=-1
  Initial_filter4 : Subsystem
  Initial_filter5 : Subsystem
  Initial_filter6 : Subsystem
  Initial_filter7 : Subsystem
  Initial_filter8 : Subsystem
  Initial_filter9 : Subsystem
  Math Function1 : Math  Operator=mod  SignedPower=on
  Math Function3 : Math  Operator=mod  SignedPower=on
  Memory6 : Memory
  Memory7 : Memory
  Mux1 : Mux  Inputs=2
  Mux2 : Mux
  PI : Subsystem  mask{Kp_PLL=2*pi*fpll, Ki_PLL=(2*pi*fpll)^2/4, IntSat_PLL=20000}
      mask prompts: Kp_PLL "Proportional (P)"; Ki_PLL "Integral (I)"; IntSat_PLL "Integrator Saturation Limit"
      mask DialogControl DescGroupVar Prompt: PLL Parameters
  Scope : Scope
  Scope1 : Scope
  Scope{7,10..12} (4 alike) : Scope  NumInputPorts=2
  State-Space : StateSpace  A=lpf_A  B=lpf_B  C=lpf_C  D=lpf_D  InitialCondition=[0,50/lpf_C(2)]
  Sum : Sum  Inputs=++|
  Sum10 : Sum  Inputs=|+-
  Sum11 : Sum  Inputs=|+-
  Sum{6..9} (4 alike) : Sum  Inputs=-+|
  Transfer Fcn : TransferFcn  Denominator=[1/(2*pi*50) 1]
  "abc -> dq (Power-Invariant)" : SimplusGT/abc -> dq (Power-Invariant)  SystemSampleTime=-1  VariantActivationTime=update diagram  AllowFlexibleInterface=on  Latency=0  AutoFrameSizeCalculation=off
      settings: SourceProductName=Simplus Grid Tool
  "abc -> dq (Power-Invariant)1" : SimplusGT/abc -> dq (Power-Invariant)  SystemSampleTime=-1  VariantActivationTime=update diagram  AllowFlexibleInterface=on  Latency=0  AutoFrameSizeCalculation=off
      settings: SourceProductName=Simplus Grid Tool
  "abc -> dq (Power-Invariant)4" : SimplusGT/abc -> dq (Power-Invariant)  SystemSampleTime=-1  VariantActivationTime=update diagram  AllowFlexibleInterface=on  Latency=0  AutoFrameSizeCalculation=off
      settings: SourceProductName=Simplus Grid Tool
  delta_idq : Scope  NumInputPorts=2
  delta_vdq : Scope  NumInputPorts=2
  id : Scope  NumInputPorts=2
  iq : Scope  NumInputPorts=2
  vd : Scope  NumInputPorts=2
  vq : Scope  NumInputPorts=2
  didq : Outport
  dvdq : Outport  Port=2
  wires:
  [vq] -> vq/1, 2nd_lpf2/1, Sum9/2
  Sum11/1 -> Scope7/2, Initial_filter9/1(original)
  Sum6/1 -> Gain5/1
  "abc -> dq (Power-Invariant)1"/1 -> Scope1/1, Demux9/1
  [theta2] -> "abc -> dq (Power-Invariant)1"/2
  Sum9/1 -> Memory7/1, Sum11/1, delta_vdq/2, Initial_filter7/1(original)
  [vd] -> 2nd_lpf3/1, vd/1, Sum8/2
  Demux9/1 -> [id]  "id"
  Sum8/1 -> Memory6/1, Sum10/1, delta_vdq/1, Initial_filter6/1(original)
  Initial_filter7/1(filtered) -> Mux2/2  "Delta_vq"
  Bus Selector169/1 -> "abc -> dq (Power-Invariant)4"/1, "abc -> dq (Power-Invariant)"/1  "<v_abc>"
  Demux9/2 -> [iq]  "iq"
  [id] -> id/1, 2nd_lpf/1, Sum6/2
  2nd_lpf/1 -> id/2, Sum6/1
  Sum10/1 -> Scope7/1, Initial_filter8/1(original)
  Memory7/1 -> Sum11/2
  Initial_filter9/1(filtered) -> Mux2/4  "dDelta_vq"
  2nd_lpf1/1 -> iq/2, Sum7/1
  Mux1/1 -> didq/1
  Memory6/1 -> Sum10/2
  Bus Selector169/2 -> "abc -> dq (Power-Invariant)1"/1  "<i_abc>"
  Sum7/1 -> Gain1/1
  Demux8/1 -> [vd]  "vd"
  Initial_filter6/1(filtered) -> Mux2/1  "Delta_vd"
  Initial_filter5/1(filtered) -> Mux1/2  "Delta_iq"
  Mux2/1 -> dvdq/1
  [iq] -> iq/1, 2nd_lpf1/1, Sum7/2
  Initial_filter4/1(filtered) -> Mux1/1  "Delta_id"
  2nd_lpf2/1 -> Sum9/1, vq/2
  Gain1/1 -> delta_idq/2, Initial_filter5/1(original)
  Demux8/2 -> [vq]  "vq"
  "abc -> dq (Power-Invariant)"/1 -> Scope/1, Demux8/1
  Initial_filter8/1(filtered) -> Mux2/3  "dDelta_vd"
  [theta2] -> "abc -> dq (Power-Invariant)"/2
  2nd_lpf3/1 -> vd/2, Sum8/1
  Gain5/1 -> delta_idq/1, Initial_filter4/1(original)
  [theta] -> "abc -> dq (Power-Invariant)4"/2
  Constant1/1 -> Math Function1/2
  Add/1 -> 2nd_lpf5/1, Scope10/1
  Discrete-Time Integrator/1 -> Math Function1/1, Add/1
  Gain2/1 -> Discrete-Time Integrator1/1  "freq"
  "abc -> dq (Power-Invariant)4"/1 -> Demux2/1
  Transfer Fcn/1 -> PI/1(e)
  Math Function1/1 -> [theta]  "theta"
  Gain/1 -> State-Space/1, Scope11/1  "freq"
  PI/1(Out) -> Gain/1, Discrete-Time Integrator/1
  Demux2/2 -> Transfer Fcn/1
  [freq_orig] -> Scope12/1
  Math Function3/1 -> [theta2]  "theta"
  2nd_lpf5/1 -> Sum/1, Scope10/2
  Sum/1 -> Math Function3/1
  State-Space/1 -> Scope12/2, [freq], Scope11/2, Gain2/1
  Constant3/1 -> Math Function3/2
  Discrete-Time Integrator1/1 -> Add/2, Sum/2  "theta"
  measurement/1 -> Bus Selector169/1
  Gain3/1 -> [freq_orig]
  Bus Selector169/3 -> Gain3/1  "<w>"

== system DEF_IEEE14_case1/uDEF1/Initial_filter4 ==
  original : Inport
  Clock1 : Clock
  Gain7 : Gain
  Gain8 : Gain  Gain=0
  Switch3 : Switch  Criteria=u2 > Threshold  Threshold=Tdef_start  SaturateOnIntegerOverflow=off  InputSameDT=off
  filtered : Outport
  wires:
  Switch3/1 -> filtered/1  "dTheta"
  original/1 -> Gain8/1, Gain7/1
  Gain7/1 -> Switch3/1
  Gain8/1 -> Switch3/3
  Clock1/1 -> Switch3/2

== system DEF_IEEE14_case1/uDEF1/Initial_filter5 ==
  original : Inport
  Clock1 : Clock
  Gain7 : Gain
  Gain8 : Gain  Gain=0
  Switch3 : Switch  Criteria=u2 > Threshold  Threshold=Tdef_start  SaturateOnIntegerOverflow=off  InputSameDT=off
  filtered : Outport
  wires:
  Switch3/1 -> filtered/1  "dTheta"
  original/1 -> Gain8/1, Gain7/1
  Gain7/1 -> Switch3/1
  Gain8/1 -> Switch3/3
  Clock1/1 -> Switch3/2

== system DEF_IEEE14_case1/uDEF1/Initial_filter6 ==
  original : Inport
  Clock1 : Clock
  Gain7 : Gain
  Gain8 : Gain  Gain=0
  Switch3 : Switch  Criteria=u2 > Threshold  Threshold=Tdef_start  SaturateOnIntegerOverflow=off  InputSameDT=off
  filtered : Outport
  wires:
  Switch3/1 -> filtered/1  "dTheta"
  original/1 -> Gain8/1, Gain7/1
  Gain7/1 -> Switch3/1
  Gain8/1 -> Switch3/3
  Clock1/1 -> Switch3/2

== system DEF_IEEE14_case1/uDEF1/Initial_filter7 ==
  original : Inport
  Clock1 : Clock
  Gain7 : Gain
  Gain8 : Gain  Gain=0
  Switch3 : Switch  Criteria=u2 > Threshold  Threshold=Tdef_start  SaturateOnIntegerOverflow=off  InputSameDT=off
  filtered : Outport
  wires:
  Switch3/1 -> filtered/1  "dTheta"
  original/1 -> Gain8/1, Gain7/1
  Gain7/1 -> Switch3/1
  Gain8/1 -> Switch3/3
  Clock1/1 -> Switch3/2

== system DEF_IEEE14_case1/uDEF1/Initial_filter8 ==
  original : Inport
  Clock1 : Clock
  Gain7 : Gain
  Gain8 : Gain  Gain=0
  Switch3 : Switch  Criteria=u2 > Threshold  Threshold=Tdef_start  SaturateOnIntegerOverflow=off  InputSameDT=off
  filtered : Outport
  wires:
  Switch3/1 -> filtered/1  "dTheta"
  original/1 -> Gain8/1, Gain7/1
  Gain7/1 -> Switch3/1
  Gain8/1 -> Switch3/3
  Clock1/1 -> Switch3/2

== system DEF_IEEE14_case1/uDEF1/Initial_filter9 ==
  original : Inport
  Clock1 : Clock
  Gain7 : Gain
  Gain8 : Gain  Gain=0
  Switch3 : Switch  Criteria=u2 > Threshold  Threshold=Tdef_start  SaturateOnIntegerOverflow=off  InputSameDT=off
  filtered : Outport
  wires:
  Switch3/1 -> filtered/1  "dTheta"
  original/1 -> Gain8/1, Gain7/1
  Gain7/1 -> Switch3/1
  Gain8/1 -> Switch3/3
  Clock1/1 -> Switch3/2

== system DEF_IEEE14_case1/uDEF1/PI ==
  e : Inport
  Discrete-Time Integrator : DiscreteIntegrator  gainval=1  InitialCondition=2*pi*Fbase  SampleTime=Ts  LimitOutput=on  UpperSaturationLimit=2*pi*Fbase + IntSat_PLL  LowerSaturationLimit=2*pi*Fbase - IntSat_PLL  ICPrevOutput=DiscIntNeverNeededParam  ICPrevScaledInput=DiscIntNeverNeededParam
  Ki : Gain  Gain=Ki_PLL  SaturateOnIntegerOverflow=on  OutDataTypeStr=Inherit: Same as input  ParamDataTypeStr=Inherit: Same as input
  Kp : Gain  Gain=Kp_PLL  SaturateOnIntegerOverflow=on  OutDataTypeStr=Inherit: Same as input  ParamDataTypeStr=Inherit: Same as input
  Sum4 : Sum  SaturateOnIntegerOverflow=on
  Out : Outport
  wires:
  Ki/1 -> Discrete-Time Integrator/1
  Kp/1 -> Sum4/1
  e/1 -> Ki/1, Kp/1
  Discrete-Time Integrator/1 -> Sum4/2
  Sum4/1 -> Out/1

== system DEF_IEEE14_case1/uDEF2/Initial_filter4 ==
  original : Inport
  Clock1 : Clock
  Gain7 : Gain
  Gain8 : Gain  Gain=0
  Switch3 : Switch  Criteria=u2 > Threshold  Threshold=Tdef_start  SaturateOnIntegerOverflow=off  InputSameDT=off
  filtered : Outport
  wires:
  Switch3/1 -> filtered/1  "dTheta"
  original/1 -> Gain8/1, Gain7/1
  Gain7/1 -> Switch3/1
  Gain8/1 -> Switch3/3
  Clock1/1 -> Switch3/2

== system DEF_IEEE14_case1/uDEF2/Initial_filter5 ==
  original : Inport
  Clock1 : Clock
  Gain7 : Gain
  Gain8 : Gain  Gain=0
  Switch3 : Switch  Criteria=u2 > Threshold  Threshold=Tdef_start  SaturateOnIntegerOverflow=off  InputSameDT=off
  filtered : Outport
  wires:
  Switch3/1 -> filtered/1  "dTheta"
  original/1 -> Gain8/1, Gain7/1
  Gain7/1 -> Switch3/1
  Gain8/1 -> Switch3/3
  Clock1/1 -> Switch3/2

== system DEF_IEEE14_case1/uDEF2/Initial_filter6 ==
  original : Inport
  Clock1 : Clock
  Gain7 : Gain
  Gain8 : Gain  Gain=0
  Switch3 : Switch  Criteria=u2 > Threshold  Threshold=Tdef_start  SaturateOnIntegerOverflow=off  InputSameDT=off
  filtered : Outport
  wires:
  Switch3/1 -> filtered/1  "dTheta"
  original/1 -> Gain8/1, Gain7/1
  Gain7/1 -> Switch3/1
  Gain8/1 -> Switch3/3
  Clock1/1 -> Switch3/2

== system DEF_IEEE14_case1/uDEF2/Initial_filter7 ==
  original : Inport
  Clock1 : Clock
  Gain7 : Gain
  Gain8 : Gain  Gain=0
  Switch3 : Switch  Criteria=u2 > Threshold  Threshold=Tdef_start  SaturateOnIntegerOverflow=off  InputSameDT=off
  filtered : Outport
  wires:
  Switch3/1 -> filtered/1  "dTheta"
  original/1 -> Gain8/1, Gain7/1
  Gain7/1 -> Switch3/1
  Gain8/1 -> Switch3/3
  Clock1/1 -> Switch3/2

== system DEF_IEEE14_case1/uDEF2/Initial_filter8 ==
  original : Inport
  Clock1 : Clock
  Gain7 : Gain
  Gain8 : Gain  Gain=0
  Switch3 : Switch  Criteria=u2 > Threshold  Threshold=Tdef_start  SaturateOnIntegerOverflow=off  InputSameDT=off
  filtered : Outport
  wires:
  Switch3/1 -> filtered/1  "dTheta"
  original/1 -> Gain8/1, Gain7/1
  Gain7/1 -> Switch3/1
  Gain8/1 -> Switch3/3
  Clock1/1 -> Switch3/2

== system DEF_IEEE14_case1/uDEF2/Initial_filter9 ==
  original : Inport
  Clock1 : Clock
  Gain7 : Gain
  Gain8 : Gain  Gain=0
  Switch3 : Switch  Criteria=u2 > Threshold  Threshold=Tdef_start  SaturateOnIntegerOverflow=off  InputSameDT=off
  filtered : Outport
  wires:
  Switch3/1 -> filtered/1  "dTheta"
  original/1 -> Gain8/1, Gain7/1
  Gain7/1 -> Switch3/1
  Gain8/1 -> Switch3/3
  Clock1/1 -> Switch3/2

== system DEF_IEEE14_case1/uDEF2/PI ==
  e : Inport
  Discrete-Time Integrator : DiscreteIntegrator  gainval=1  InitialCondition=2*pi*Fbase  SampleTime=Ts  LimitOutput=on  UpperSaturationLimit=2*pi*Fbase + IntSat_PLL  LowerSaturationLimit=2*pi*Fbase - IntSat_PLL  ICPrevOutput=DiscIntNeverNeededParam  ICPrevScaledInput=DiscIntNeverNeededParam
  Ki : Gain  Gain=Ki_PLL  SaturateOnIntegerOverflow=on  OutDataTypeStr=Inherit: Same as input  ParamDataTypeStr=Inherit: Same as input
  Kp : Gain  Gain=Kp_PLL  SaturateOnIntegerOverflow=on  OutDataTypeStr=Inherit: Same as input  ParamDataTypeStr=Inherit: Same as input
  Sum4 : Sum  SaturateOnIntegerOverflow=on
  Out : Outport
  wires:
  Ki/1 -> Discrete-Time Integrator/1
  Kp/1 -> Sum4/1
  e/1 -> Ki/1, Kp/1
  Discrete-Time Integrator/1 -> Sum4/2
  Sum4/1 -> Out/1

== system DEF_IEEE14_case1/uDEF3/Initial_filter4 ==
  original : Inport
  Clock1 : Clock
  Gain7 : Gain
  Gain8 : Gain  Gain=0
  Switch3 : Switch  Criteria=u2 > Threshold  Threshold=Tdef_start  SaturateOnIntegerOverflow=off  InputSameDT=off
  filtered : Outport
  wires:
  Clock1/1 -> Switch3/2
  Gain8/1 -> Switch3/3
  Gain7/1 -> Switch3/1
  original/1 -> Gain7/1, Gain8/1
  Switch3/1 -> filtered/1  "dTheta"

== system DEF_IEEE14_case1/uDEF3/Initial_filter5 ==
  original : Inport
  Clock1 : Clock
  Gain7 : Gain
  Gain8 : Gain  Gain=0
  Switch3 : Switch  Criteria=u2 > Threshold  Threshold=Tdef_start  SaturateOnIntegerOverflow=off  InputSameDT=off
  filtered : Outport
  wires:
  Clock1/1 -> Switch3/2
  Gain8/1 -> Switch3/3
  Gain7/1 -> Switch3/1
  original/1 -> Gain7/1, Gain8/1
  Switch3/1 -> filtered/1  "dTheta"

== system DEF_IEEE14_case1/uDEF3/Initial_filter6 ==
  original : Inport
  Clock1 : Clock
  Gain7 : Gain
  Gain8 : Gain  Gain=0
  Switch3 : Switch  Criteria=u2 > Threshold  Threshold=Tdef_start  SaturateOnIntegerOverflow=off  InputSameDT=off
  filtered : Outport
  wires:
  Clock1/1 -> Switch3/2
  Gain8/1 -> Switch3/3
  Gain7/1 -> Switch3/1
  original/1 -> Gain7/1, Gain8/1
  Switch3/1 -> filtered/1  "dTheta"

== system DEF_IEEE14_case1/uDEF3/Initial_filter7 ==
  original : Inport
  Clock1 : Clock
  Gain7 : Gain
  Gain8 : Gain  Gain=0
  Switch3 : Switch  Criteria=u2 > Threshold  Threshold=Tdef_start  SaturateOnIntegerOverflow=off  InputSameDT=off
  filtered : Outport
  wires:
  Clock1/1 -> Switch3/2
  Gain8/1 -> Switch3/3
  Gain7/1 -> Switch3/1
  original/1 -> Gain7/1, Gain8/1
  Switch3/1 -> filtered/1  "dTheta"

== system DEF_IEEE14_case1/uDEF3/Initial_filter8 ==
  original : Inport
  Clock1 : Clock
  Gain7 : Gain
  Gain8 : Gain  Gain=0
  Switch3 : Switch  Criteria=u2 > Threshold  Threshold=Tdef_start  SaturateOnIntegerOverflow=off  InputSameDT=off
  filtered : Outport
  wires:
  Clock1/1 -> Switch3/2
  Gain8/1 -> Switch3/3
  Gain7/1 -> Switch3/1
  original/1 -> Gain7/1, Gain8/1
  Switch3/1 -> filtered/1  "dTheta"

== system DEF_IEEE14_case1/uDEF3/Initial_filter9 ==
  original : Inport
  Clock1 : Clock
  Gain7 : Gain
  Gain8 : Gain  Gain=0
  Switch3 : Switch  Criteria=u2 > Threshold  Threshold=Tdef_start  SaturateOnIntegerOverflow=off  InputSameDT=off
  filtered : Outport
  wires:
  Clock1/1 -> Switch3/2
  Gain8/1 -> Switch3/3
  Gain7/1 -> Switch3/1
  original/1 -> Gain7/1, Gain8/1
  Switch3/1 -> filtered/1  "dTheta"

== system DEF_IEEE14_case1/uDEF3/PI ==
  e : Inport
  Discrete-Time Integrator : DiscreteIntegrator  gainval=1  InitialCondition=2*pi*Fbase  SampleTime=Ts  LimitOutput=on  UpperSaturationLimit=2*pi*Fbase + IntSat_PLL  LowerSaturationLimit=2*pi*Fbase - IntSat_PLL  ICPrevOutput=DiscIntNeverNeededParam  ICPrevScaledInput=DiscIntNeverNeededParam
  Ki : Gain  Gain=Ki_PLL  SaturateOnIntegerOverflow=on  OutDataTypeStr=Inherit: Same as input  ParamDataTypeStr=Inherit: Same as input
  Kp : Gain  Gain=Kp_PLL  SaturateOnIntegerOverflow=on  OutDataTypeStr=Inherit: Same as input  ParamDataTypeStr=Inherit: Same as input
  Sum4 : Sum  SaturateOnIntegerOverflow=on
  Out : Outport
  wires:
  Sum4/1 -> Out/1
  Discrete-Time Integrator/1 -> Sum4/2
  e/1 -> Kp/1, Ki/1
  Kp/1 -> Sum4/1
  Ki/1 -> Discrete-Time Integrator/1

== system DEF_IEEE14_case1/uDEF5/Initial_filter4 ==
  original : Inport
  Clock1 : Clock
  Gain7 : Gain
  Gain8 : Gain  Gain=0
  Switch3 : Switch  Criteria=u2 > Threshold  Threshold=Tdef_start  SaturateOnIntegerOverflow=off  InputSameDT=off
  filtered : Outport
  wires:
  Switch3/1 -> filtered/1  "dTheta"
  original/1 -> Gain8/1, Gain7/1
  Gain7/1 -> Switch3/1
  Gain8/1 -> Switch3/3
  Clock1/1 -> Switch3/2

== system DEF_IEEE14_case1/uDEF5/Initial_filter5 ==
  original : Inport
  Clock1 : Clock
  Gain7 : Gain
  Gain8 : Gain  Gain=0
  Switch3 : Switch  Criteria=u2 > Threshold  Threshold=Tdef_start  SaturateOnIntegerOverflow=off  InputSameDT=off
  filtered : Outport
  wires:
  Switch3/1 -> filtered/1  "dTheta"
  original/1 -> Gain8/1, Gain7/1
  Gain7/1 -> Switch3/1
  Gain8/1 -> Switch3/3
  Clock1/1 -> Switch3/2

== system DEF_IEEE14_case1/uDEF5/Initial_filter6 ==
  original : Inport
  Clock1 : Clock
  Gain7 : Gain
  Gain8 : Gain  Gain=0
  Switch3 : Switch  Criteria=u2 > Threshold  Threshold=Tdef_start  SaturateOnIntegerOverflow=off  InputSameDT=off
  filtered : Outport
  wires:
  Switch3/1 -> filtered/1  "dTheta"
  original/1 -> Gain8/1, Gain7/1
  Gain7/1 -> Switch3/1
  Gain8/1 -> Switch3/3
  Clock1/1 -> Switch3/2

== system DEF_IEEE14_case1/uDEF5/Initial_filter7 ==
  original : Inport
  Clock1 : Clock
  Gain7 : Gain
  Gain8 : Gain  Gain=0
  Switch3 : Switch  Criteria=u2 > Threshold  Threshold=Tdef_start  SaturateOnIntegerOverflow=off  InputSameDT=off
  filtered : Outport
  wires:
  Switch3/1 -> filtered/1  "dTheta"
  original/1 -> Gain8/1, Gain7/1
  Gain7/1 -> Switch3/1
  Gain8/1 -> Switch3/3
  Clock1/1 -> Switch3/2

== system DEF_IEEE14_case1/uDEF5/Initial_filter8 ==
  original : Inport
  Clock1 : Clock
  Gain7 : Gain
  Gain8 : Gain  Gain=0
  Switch3 : Switch  Criteria=u2 > Threshold  Threshold=Tdef_start  SaturateOnIntegerOverflow=off  InputSameDT=off
  filtered : Outport
  wires:
  Switch3/1 -> filtered/1  "dTheta"
  original/1 -> Gain8/1, Gain7/1
  Gain7/1 -> Switch3/1
  Gain8/1 -> Switch3/3
  Clock1/1 -> Switch3/2

== system DEF_IEEE14_case1/uDEF5/Initial_filter9 ==
  original : Inport
  Clock1 : Clock
  Gain7 : Gain
  Gain8 : Gain  Gain=0
  Switch3 : Switch  Criteria=u2 > Threshold  Threshold=Tdef_start  SaturateOnIntegerOverflow=off  InputSameDT=off
  filtered : Outport
  wires:
  Switch3/1 -> filtered/1  "dTheta"
  original/1 -> Gain8/1, Gain7/1
  Gain7/1 -> Switch3/1
  Gain8/1 -> Switch3/3
  Clock1/1 -> Switch3/2
